simulink model "Commande"  (R2020b)
settings: Solver=VariableStepAuto  StartTime=0.0  StopTime=1  RelTol=1e-3
undefined symbols (not defined in the file or in its folder): FC, FuelCellLoadFcn, gcbh, ln, sps_rtmsupport, Ts
libraries: simulink x43, powerlib x37, powerlib_meascontrol x7, fuzblock x4, powerlib_extras x2
(part 3 of 3)

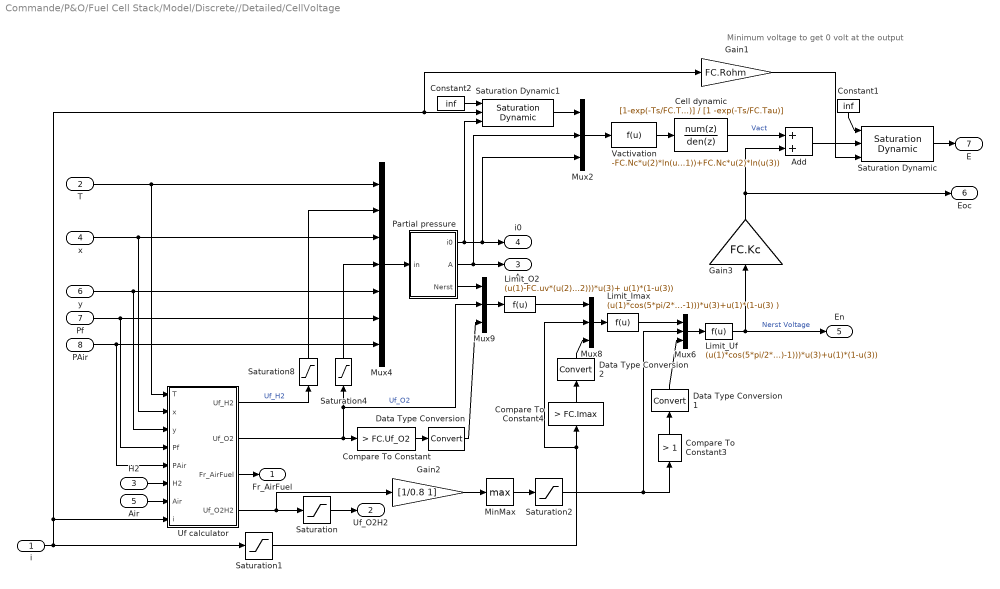
== system Commande/P&O/Fuel Cell Stack/Model/Discrete//Detailed/CellVoltage ==
  note: Minimum voltage to get 0 volt at the output
  i : Inport
  T : Inport  Port=2
  H2 : Inport  Port=3
  x : Inport  Port=4
  Air : Inport  Port=5
  y : Inport  Port=6
  Pf : Inport  Port=7
  PAir : Inport  Port=8
  Add : Sum
  Cell dynamic : DiscreteTransferFcn  Numerator=[1-exp(-Ts/FC.Tau)]  Denominator=[1 -exp(-Ts/FC.Tau)]  SampleTime=Ts
  Compare To Constant : simulink/Logic and Bit Operations/Compare To Constant  relop=>  const=FC.Uf_O2  OutDataTypeStr=boolean
  Compare To Constant3 : simulink/Logic and Bit Operations/Compare To Constant  relop=>  const=1  OutDataTypeStr=boolean
  Compare To Constant4 : simulink/Logic and Bit Operations/Compare To Constant  relop=>  const=FC.Imax  OutDataTypeStr=boolean
  Constant1 : Constant  Value=inf
  Constant2 : Constant  Value=inf
  Data Type Conversion : DataTypeConversion
  Data Type Conversion1 : DataTypeConversion
  Data Type Conversion2 : DataTypeConversion
  Gain1 : Gain  Gain=FC.Rohm
  Gain2 : Gain  Gain=[1/0.8 1]
  Gain3 : Gain  Gain=FC.Kc
  Limit_Imax : Fcn  Expr=(u(1)*cos(5*pi/2*(u(2)/FC.Imax-1)))*u(3)+u(1)*(1-u(3) )
  Limit_O2 : Fcn  Expr=(u(1)-FC.uv*(u(2)-FC.Uf_O2)/(FC.Kc*(FC.ufO2max-FC.Uf_O2)))*u(3)+ u(1)*(1-u(3))
  Limit_Uf : Fcn  Expr=(u(1)*cos(5*pi/2*(u(2)-1)))*u(3)+u(1)*(1-u(3))
  MinMax : MinMax  Function=max
  Mux{2,6,8..9} (4 alike) : Mux  Inputs=3
  Mux4 : Mux  Inputs=7
  Partial pressure : Subsystem
  Saturation : Saturate  UpperLimit=0.9999  LowerLimit=0.0001
  Saturation Dynamic : simulink/Discontinuities/Saturation Dynamic  OutMin=[]  OutMax=[]  OutDataTypeStr=Inherit: Same as second input  OutDataType=fixdt(1, 16)  OutScaling=2^-10  DoSatur=off
  Saturation Dynamic1 : simulink/Discontinuities/Saturation Dynamic  OutMin=[]  OutMax=[]  OutDataTypeStr=Inherit: Same as second input  OutDataType=fixdt(1, 16)  OutScaling=2^-10  DoSatur=off
  Saturation1 : Saturate  UpperLimit=FC.Imax*1.2  LowerLimit=0
  Saturation2 : Saturate  UpperLimit=1.2  LowerLimit=0
  Saturation4 : Saturate  UpperLimit=FC.Uf_O2  LowerLimit=0
  Saturation8 : Saturate  UpperLimit=FC.Uf_H2  LowerLimit=0
  Uf calculator : Subsystem
  Vactivation : Fcn  Expr=-FC.Nc*u(2)*ln(u(1))+FC.Nc*u(2)*ln(u(3))
  Fr_AirFuel : Outport  VectorParamsAs1DForOutWhenUnconnected=off
  Uf_O2H2 : Outport  Port=2  VectorParamsAs1DForOutWhenUnconnected=off
  A : Outport  Port=3  VectorParamsAs1DForOutWhenUnconnected=off
  i0 : Outport  Port=4  VectorParamsAs1DForOutWhenUnconnected=off
  En : Outport  Port=5  VectorParamsAs1DForOutWhenUnconnected=off
  Eoc : Outport  Port=6  VectorParamsAs1DForOutWhenUnconnected=off
  E : Outport  Port=7  VectorParamsAs1DForOutWhenUnconnected=off
  wires:
  Gain3/1 -> Eoc/1, Add/2
  T/1 -> Uf calculator/1(T), Mux4/1
  x/1 -> Mux4/3, Uf calculator/2(x)
  y/1 -> Mux4/5, Uf calculator/3(y)
  Pf/1 -> Mux4/6, Uf calculator/4(Pf)
  PAir/1 -> Mux4/7, Uf calculator/5(PAir)
  Partial pressure/1(i0) -> Saturation Dynamic1/3, i0/1, Mux2/3
  Partial pressure/2(A) -> A/1, Mux2/2
  H2/1 -> Uf calculator/6(H2)
  i/1 -> Uf calculator/8(i), Saturation Dynamic1/2, Gain1/1, Saturation1/1
  Uf calculator/1(Uf_H2) -> Saturation8/1  "Uf_H2"
  Uf calculator/2(Uf_O2) -> Compare To Constant/1, Saturation4/1, Mux9/2  "Uf_O2"
  Air/1 -> Uf calculator/7(Air)
  Mux8/1 -> Limit_Imax/1
  Limit_Imax/1 -> Mux6/1
  Limit_Uf/1 -> Gain3/1, En/1  "Nerst Voltage"
  Uf calculator/3(Fr_AirFuel) -> Fr_AirFuel/1
  Mux9/1 -> Limit_O2/1
  Limit_O2/1 -> Mux8/1
  Saturation8/1 -> Mux4/2
  Uf calculator/4(Uf_O2H2) -> Saturation/1, Gain2/1
  Mux4/1 -> Partial pressure/1(in)
  Constant2/1 -> Saturation Dynamic1/1
  Saturation Dynamic1/1 -> Mux2/1
  Mux2/1 -> Vactivation/1
  Vactivation/1 -> Cell dynamic/1
  Cell dynamic/1 -> Add/1  "Vact"
  Add/1 -> Saturation Dynamic/2
  Saturation Dynamic/1 -> E/1
  Constant1/1 -> Saturation Dynamic/1
  Gain1/1 -> Saturation Dynamic/3
  Mux6/1 -> Limit_Uf/1
  Saturation/1 -> Uf_O2H2/1
  MinMax/1 -> Saturation2/1
  Saturation4/1 -> Mux4/4
  Partial pressure/3(Nerst) -> Mux9/1
  Gain2/1 -> MinMax/1
  Compare To Constant/1 -> Data Type Conversion/1
  Data Type Conversion/1 -> Mux9/3
  Data Type Conversion2/1 -> Mux8/3
  Compare To Constant4/1 -> Data Type Conversion2/1
  Saturation1/1 -> Mux8/2, Compare To Constant4/1
  Saturation2/1 -> Mux6/2, Compare To Constant3/1
  Compare To Constant3/1 -> Data Type Conversion1/1
  Data Type Conversion1/1 -> Mux6/3

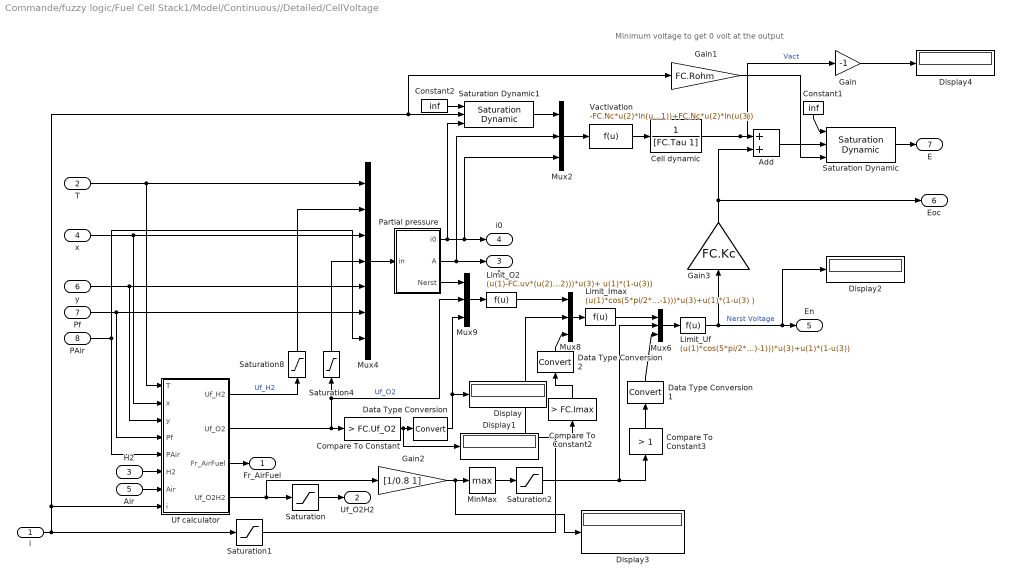
== system Commande/fuzzy logic/Fuel Cell Stack1/Model/Continuous//Detailed/CellVoltage ==
  note: Minimum voltage to get 0 volt at the output
  i : Inport
  T : Inport  Port=2
  H2 : Inport  Port=3
  x : Inport  Port=4
  Air : Inport  Port=5
  y : Inport  Port=6
  Pf : Inport  Port=7
  PAir : Inport  Port=8
  Add : Sum
  Cell dynamic : TransferFcn  Denominator=[FC.Tau 1]
  Compare To Constant : simulink/Logic and Bit Operations/Compare To Constant  relop=>  const=FC.Uf_O2  OutDataTypeStr=boolean
  Compare To Constant2 : simulink/Logic and Bit Operations/Compare To Constant  relop=>  const=FC.Imax  OutDataTypeStr=boolean
  Compare To Constant3 : simulink/Logic and Bit Operations/Compare To Constant  relop=>  const=1  OutDataTypeStr=boolean
  Constant1 : Constant  Value=inf
  Constant2 : Constant  Value=inf
  Data Type Conversion : DataTypeConversion
  Data Type Conversion1 : DataTypeConversion
  Data Type Conversion2 : DataTypeConversion
  Display{,1..4} (5 alike) : Display
  Gain : Gain  Gain=-1
  Gain1 : Gain  Gain=FC.Rohm
  Gain2 : Gain  Gain=[1/0.8 1]
  Gain3 : Gain  Gain=FC.Kc
  Limit_Imax : Fcn  Expr=(u(1)*cos(5*pi/2*(u(2)/FC.Imax-1)))*u(3)+u(1)*(1-u(3) )
  Limit_O2 : Fcn  Expr=(u(1)-FC.uv*(u(2)-FC.Uf_O2)/(FC.Kc*(FC.ufO2max-FC.Uf_O2)))*u(3)+ u(1)*(1-u(3))
  Limit_Uf : Fcn  Expr=(u(1)*cos(5*pi/2*(u(2)-1)))*u(3)+u(1)*(1-u(3))
  MinMax : MinMax  Function=max
  Mux{2,6,8..9} (4 alike) : Mux  Inputs=3
  Mux4 : Mux  Inputs=7
  Partial pressure : Subsystem
  Saturation : Saturate  UpperLimit=0.9999  LowerLimit=0.0001
  Saturation Dynamic : simulink/Discontinuities/Saturation Dynamic  OutMin=[]  OutMax=[]  OutDataTypeStr=Inherit: Same as second input  OutDataType=fixdt(1, 16)  OutScaling=2^-10  DoSatur=off
  Saturation Dynamic1 : simulink/Discontinuities/Saturation Dynamic  OutMin=[]  OutMax=[]  OutDataTypeStr=Inherit: Same as second input  OutDataType=fixdt(1, 16)  OutScaling=2^-10  DoSatur=off
  Saturation1 : Saturate  UpperLimit=FC.Imax*1.2  LowerLimit=0
  Saturation2 : Saturate  UpperLimit=1.2  LowerLimit=0
  Saturation4 : Saturate  UpperLimit=FC.Uf_O2  LowerLimit=0
  Saturation8 : Saturate  UpperLimit=FC.Uf_H2  LowerLimit=0
  Uf calculator : Subsystem
  Vactivation : Fcn  Expr=-FC.Nc*u(2)*ln(u(1))+FC.Nc*u(2)*ln(u(3))
  Fr_AirFuel : Outport  VectorParamsAs1DForOutWhenUnconnected=off
  Uf_O2H2 : Outport  Port=2  VectorParamsAs1DForOutWhenUnconnected=off
  A : Outport  Port=3  VectorParamsAs1DForOutWhenUnconnected=off
  i0 : Outport  Port=4  VectorParamsAs1DForOutWhenUnconnected=off
  En : Outport  Port=5  VectorParamsAs1DForOutWhenUnconnected=off
  Eoc : Outport  Port=6  VectorParamsAs1DForOutWhenUnconnected=off
  E : Outport  Port=7  VectorParamsAs1DForOutWhenUnconnected=off
  wires:
  Gain3/1 -> Eoc/1, Add/2
  Data Type Conversion1/1 -> Mux6/3
  Compare To Constant3/1 -> Data Type Conversion1/1
  Saturation2/1 -> Mux6/2, Compare To Constant3/1
  Saturation1/1 -> Mux8/2, Compare To Constant2/1
  Compare To Constant2/1 -> Data Type Conversion2/1
  Data Type Conversion2/1 -> Mux8/3
  Compare To Constant/1 -> Display1/1, Data Type Conversion/1
  Gain2/1 -> Display3/1, MinMax/1
  Partial pressure/3(Nerst) -> Mux9/1
  Saturation4/1 -> Mux4/4
  MinMax/1 -> Saturation2/1
  Saturation/1 -> Uf_O2H2/1
  Mux6/1 -> Limit_Uf/1
  Gain1/1 -> Saturation Dynamic/3
  Constant1/1 -> Saturation Dynamic/1
  Saturation Dynamic/1 -> E/1
  Add/1 -> Saturation Dynamic/2
  Cell dynamic/1 -> Gain/1, Add/1  "Vact"
  Vactivation/1 -> Cell dynamic/1
  Mux2/1 -> Vactivation/1
  Saturation Dynamic1/1 -> Mux2/1
  Constant2/1 -> Saturation Dynamic1/1
  Mux4/1 -> Partial pressure/1(in)
  Uf calculator/4(Uf_O2H2) -> Gain2/1, Saturation/1
  Saturation8/1 -> Mux4/2
  Limit_O2/1 -> Mux8/1
  Mux9/1 -> Limit_O2/1
  Uf calculator/3(Fr_AirFuel) -> Fr_AirFuel/1
  Limit_Uf/1 -> Gain3/1, Display2/1, En/1  "Nerst Voltage"
  Limit_Imax/1 -> Mux6/1
  Mux8/1 -> Limit_Imax/1
  Air/1 -> Uf calculator/7(Air)
  Uf calculator/2(Uf_O2) -> Mux9/2, Saturation4/1, Compare To Constant/1  "Uf_O2"
  Uf calculator/1(Uf_H2) -> Saturation8/1  "Uf_H2"
  i/1 -> Saturation1/1, Uf calculator/8(i), Gain1/1, Saturation Dynamic1/2
  H2/1 -> Uf calculator/6(H2)
  Partial pressure/2(A) -> Mux2/2, A/1
  Partial pressure/1(i0) -> Mux2/3, i0/1, Saturation Dynamic1/3
  PAir/1 -> Uf calculator/5(PAir), Mux4/7
  Pf/1 -> Uf calculator/4(Pf), Mux4/6
  y/1 -> Uf calculator/3(y), Mux4/5
  x/1 -> Uf calculator/2(x), Mux4/3
  T/1 -> Uf calculator/1(T), Mux4/1
  Data Type Conversion/1 -> Display/1, Mux9/3
  Gain/1 -> Display4/1

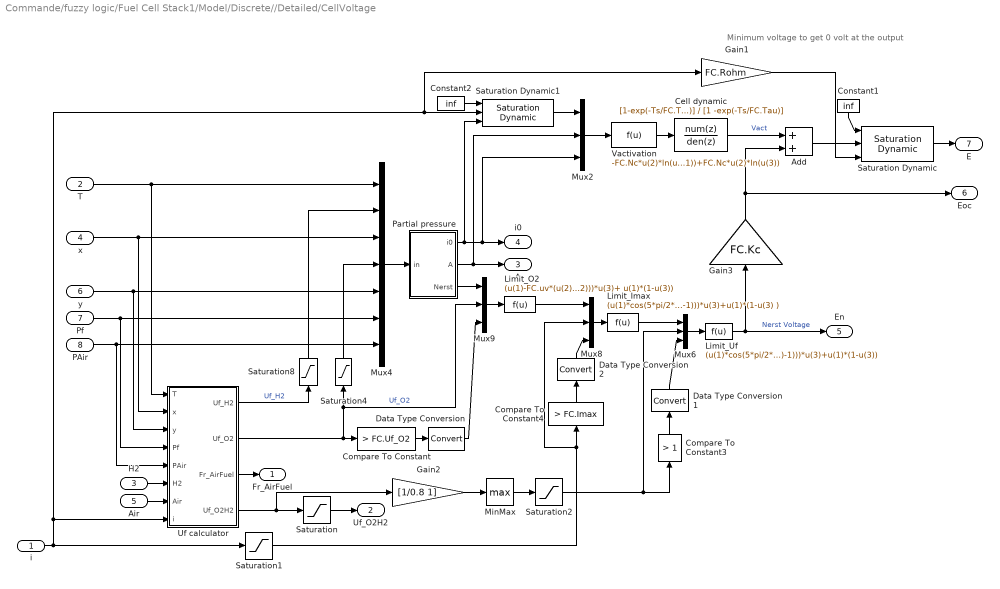
== system Commande/fuzzy logic/Fuel Cell Stack1/Model/Discrete//Detailed/CellVoltage ==
  note: Minimum voltage to get 0 volt at the output
  i : Inport
  T : Inport  Port=2
  H2 : Inport  Port=3
  x : Inport  Port=4
  Air : Inport  Port=5
  y : Inport  Port=6
  Pf : Inport  Port=7
  PAir : Inport  Port=8
  Add : Sum
  Cell dynamic : DiscreteTransferFcn  Numerator=[1-exp(-Ts/FC.Tau)]  Denominator=[1 -exp(-Ts/FC.Tau)]  SampleTime=Ts
  Compare To Constant : simulink/Logic and Bit Operations/Compare To Constant  relop=>  const=FC.Uf_O2  OutDataTypeStr=boolean
  Compare To Constant3 : simulink/Logic and Bit Operations/Compare To Constant  relop=>  const=1  OutDataTypeStr=boolean
  Compare To Constant4 : simulink/Logic and Bit Operations/Compare To Constant  relop=>  const=FC.Imax  OutDataTypeStr=boolean
  Constant1 : Constant  Value=inf
  Constant2 : Constant  Value=inf
  Data Type Conversion : DataTypeConversion
  Data Type Conversion1 : DataTypeConversion
  Data Type Conversion2 : DataTypeConversion
  Gain1 : Gain  Gain=FC.Rohm
  Gain2 : Gain  Gain=[1/0.8 1]
  Gain3 : Gain  Gain=FC.Kc
  Limit_Imax : Fcn  Expr=(u(1)*cos(5*pi/2*(u(2)/FC.Imax-1)))*u(3)+u(1)*(1-u(3) )
  Limit_O2 : Fcn  Expr=(u(1)-FC.uv*(u(2)-FC.Uf_O2)/(FC.Kc*(FC.ufO2max-FC.Uf_O2)))*u(3)+ u(1)*(1-u(3))
  Limit_Uf : Fcn  Expr=(u(1)*cos(5*pi/2*(u(2)-1)))*u(3)+u(1)*(1-u(3))
  MinMax : MinMax  Function=max
  Mux{2,6,8..9} (4 alike) : Mux  Inputs=3
  Mux4 : Mux  Inputs=7
  Partial pressure : Subsystem
  Saturation : Saturate  UpperLimit=0.9999  LowerLimit=0.0001
  Saturation Dynamic : simulink/Discontinuities/Saturation Dynamic  OutMin=[]  OutMax=[]  OutDataTypeStr=Inherit: Same as second input  OutDataType=fixdt(1, 16)  OutScaling=2^-10  DoSatur=off
  Saturation Dynamic1 : simulink/Discontinuities/Saturation Dynamic  OutMin=[]  OutMax=[]  OutDataTypeStr=Inherit: Same as second input  OutDataType=fixdt(1, 16)  OutScaling=2^-10  DoSatur=off
  Saturation1 : Saturate  UpperLimit=FC.Imax*1.2  LowerLimit=0
  Saturation2 : Saturate  UpperLimit=1.2  LowerLimit=0
  Saturation4 : Saturate  UpperLimit=FC.Uf_O2  LowerLimit=0
  Saturation8 : Saturate  UpperLimit=FC.Uf_H2  LowerLimit=0
  Uf calculator : Subsystem
  Vactivation : Fcn  Expr=-FC.Nc*u(2)*ln(u(1))+FC.Nc*u(2)*ln(u(3))
  Fr_AirFuel : Outport  VectorParamsAs1DForOutWhenUnconnected=off
  Uf_O2H2 : Outport  Port=2  VectorParamsAs1DForOutWhenUnconnected=off
  A : Outport  Port=3  VectorParamsAs1DForOutWhenUnconnected=off
  i0 : Outport  Port=4  VectorParamsAs1DForOutWhenUnconnected=off
  En : Outport  Port=5  VectorParamsAs1DForOutWhenUnconnected=off
  Eoc : Outport  Port=6  VectorParamsAs1DForOutWhenUnconnected=off
  E : Outport  Port=7  VectorParamsAs1DForOutWhenUnconnected=off
  wires:
  Gain3/1 -> Eoc/1, Add/2
  T/1 -> Uf calculator/1(T), Mux4/1
  x/1 -> Mux4/3, Uf calculator/2(x)
  y/1 -> Mux4/5, Uf calculator/3(y)
  Pf/1 -> Mux4/6, Uf calculator/4(Pf)
  PAir/1 -> Mux4/7, Uf calculator/5(PAir)
  Partial pressure/1(i0) -> Saturation Dynamic1/3, i0/1, Mux2/3
  Partial pressure/2(A) -> A/1, Mux2/2
  H2/1 -> Uf calculator/6(H2)
  i/1 -> Uf calculator/8(i), Saturation Dynamic1/2, Gain1/1, Saturation1/1
  Uf calculator/1(Uf_H2) -> Saturation8/1  "Uf_H2"
  Uf calculator/2(Uf_O2) -> Compare To Constant/1, Saturation4/1, Mux9/2  "Uf_O2"
  Air/1 -> Uf calculator/7(Air)
  Mux8/1 -> Limit_Imax/1
  Limit_Imax/1 -> Mux6/1
  Limit_Uf/1 -> Gain3/1, En/1  "Nerst Voltage"
  Uf calculator/3(Fr_AirFuel) -> Fr_AirFuel/1
  Mux9/1 -> Limit_O2/1
  Limit_O2/1 -> Mux8/1
  Saturation8/1 -> Mux4/2
  Uf calculator/4(Uf_O2H2) -> Saturation/1, Gain2/1
  Mux4/1 -> Partial pressure/1(in)
  Constant2/1 -> Saturation Dynamic1/1
  Saturation Dynamic1/1 -> Mux2/1
  Mux2/1 -> Vactivation/1
  Vactivation/1 -> Cell dynamic/1
  Cell dynamic/1 -> Add/1  "Vact"
  Add/1 -> Saturation Dynamic/2
  Saturation Dynamic/1 -> E/1
  Constant1/1 -> Saturation Dynamic/1
  Gain1/1 -> Saturation Dynamic/3
  Mux6/1 -> Limit_Uf/1
  Saturation/1 -> Uf_O2H2/1
  MinMax/1 -> Saturation2/1
  Saturation4/1 -> Mux4/4
  Partial pressure/3(Nerst) -> Mux9/1
  Gain2/1 -> MinMax/1
  Compare To Constant/1 -> Data Type Conversion/1
  Data Type Conversion/1 -> Mux9/3
  Data Type Conversion2/1 -> Mux8/3
  Compare To Constant4/1 -> Data Type Conversion2/1
  Saturation1/1 -> Mux8/2, Compare To Constant4/1
  Saturation2/1 -> Mux6/2, Compare To Constant3/1
  Compare To Constant3/1 -> Data Type Conversion1/1
  Data Type Conversion1/1 -> Mux6/3

== system Commande/INC 1/Fuel Cell Stack/Model/Continuous//Detailed/CellVoltage/Partial pressure ==
  in : Inport
  A2 : Fcn  Expr=(FC.R*u(1))/(2*FC.alpha*FC.F)
  Constant : Constant
  Cr : Fcn  Expr=(u(2)*FC.Pstd+u(3)*FC.Pstd)/(FC.R*u(1))
  Display : Display
  Display1 : Display
  Mux1 : Mux  Inputs=2
  Mux2 : Mux
  Nerst Voltage : Fcn  Expr=1.229+(u(1)-298.15)*(-44.43/(FC.z*FC.F))+(FC.R*u(1)/(FC.z*FC.F))*(log(u(2)*sqrt(u(3))/u(4)))
  PH2 : Fcn  Expr=u(3)*(1-u(2))*u(6)
  PH2O : Fcn  Expr=(FC.xy+2*u(5)*u(4))*u(7)
  PO2 : Fcn  Expr=u(5)*(1-u(4))*u(7)
  Saturation1 : Saturate  UpperLimit=inf  LowerLimit=0.0001
  Saturation4 : Saturate  UpperLimit=inf  LowerLimit=0.0001
  Saturation5 : Saturate  UpperLimit=inf  LowerLimit=0.0001
  Switch : Switch  Threshold=273+100
  Temp : Fcn  Expr=u(1)
  i0 calc : Fcn  Expr=2*FC.F*FC.k*u(1)*u(2)*exp(-FC.Dg/(FC.R*u(1)))/FC.h
  i0 : Outport  VectorParamsAs1DForOutWhenUnconnected=off
  A : Outport  Port=2  VectorParamsAs1DForOutWhenUnconnected=off
  Nerst : Outport  Port=3  VectorParamsAs1DForOutWhenUnconnected=off
  wires:
  Temp/1 -> Mux2/1, Switch/2, A2/1, Mux1/1
  i0 calc/1 -> i0/1
  Nerst Voltage/1 -> Display1/1, Nerst/1
  A2/1 -> A/1
  PH2O/1 -> Saturation5/1
  PO2/1 -> Saturation4/1
  PH2/1 -> Saturation1/1
  Saturation1/1 -> Mux2/2
  Saturation4/1 -> Mux2/3
  Switch/1 -> Mux2/4
  Saturation5/1 -> Switch/1
  Constant/1 -> Switch/3
  Mux2/1 -> Nerst Voltage/1, Cr/1
  in/1 -> PH2O/1, Display/1, Temp/1, PH2/1, PO2/1
  Mux1/1 -> i0 calc/1
  Cr/1 -> Mux1/2

== system Commande/INC 1/Fuel Cell Stack/Model/Continuous//Detailed/CellVoltage/Uf calculator ==
  T : Inport
  x : Inport  Port=2
  y : Inport  Port=3
  Pf : Inport  Port=4
  PAir : Inport  Port=5
  H2 : Inport  Port=6
  Air : Inport  Port=7
  i : Inport  Port=8
  AIR_flow_rate : Display
  Compare To Zero : simulink/Logic and Bit Operations/Compare To Zero  relop=>  OutDataTypeStr=uint8
  Constant : Constant  Value=FC.R
  Constant1 : Constant  Value=FC.sel_UfH2
  Constant2 : Constant  Value=FC.sel_UfO2
  Gain : Gain
  H2 utilization Fuel flowrate : Fcn  Expr=60000*FC.Nc*u(2)*FC.R*u(5)/(FC.z*FC.F*u(4)*FC.Pstd*u(3)*u(1))
  H2_airflow1 : Display
  Mux1 : Mux  Inputs=5
  Mux5 : Mux  Inputs=5
  Mux6 : Mux  Inputs=2
  Mux7 : Mux  Inputs=2
  O2 utilization Air flowrate : Fcn  Expr=60000*FC.Nc*u(2)*FC.R*u(5)/(4*FC.F*u(4)*FC.Pstd*u(3)*u(1))
  P_air : Display
  P_fuel : Display
  Product2 : Product  RndMeth=Zero
  Saturation3 : Saturate  UpperLimit=inf  LowerLimit=FC.AirFr_Max*0.01
  Switch{1..4} (4 alike) : Switch  Criteria=u2 > Threshold  Threshold=0.5
  UF_H2 : Display
  UF_O2 : Display
  X : Display
  Y : Display
  i_current : Display
  i_current1 : Display
  i_current2 : Display
  Uf_H2 : Outport  VectorParamsAs1DForOutWhenUnconnected=off
  Uf_O2 : Outport  Port=2  VectorParamsAs1DForOutWhenUnconnected=off
  Fr_AirFuel : Outport  Port=3  VectorParamsAs1DForOutWhenUnconnected=off
  Uf_O2H2 : Outport  Port=4  VectorParamsAs1DForOutWhenUnconnected=off
  wires:
  Switch1/1 -> Mux7/2, UF_H2/1, Uf_H2/1
  Saturation3/1 -> Mux5/3
  Switch2/1 -> Mux7/1, UF_O2/1, Uf_O2/1  "Uf_O2"
  Gain/1 -> Fr_AirFuel/1
  Switch4/1 -> Mux6/1
  Switch3/1 -> Mux6/2
  Mux6/1 -> Gain/1
  Pf/1 -> P_fuel/1, Mux1/4
  T/1 -> i_current2/1, Mux1/5, Mux5/5
  O2 utilization Air flowrate/1 -> Switch4/1, Switch2/3
  Constant2/1 -> Switch2/2, Switch4/2
  Constant1/1 -> Switch3/2, Switch1/2
  H2 utilization Fuel flowrate/1 -> Switch3/1, Switch1/3
  i/1 -> i_current/1, Compare To Zero/1, Mux1/2, i_current1/1, Mux5/2
  Air/1 -> AIR_flow_rate/1, Switch2/1, Switch4/3, Saturation3/1
  y/1 -> Y/1, Mux5/1
  H2/1 -> H2_airflow1/1, Mux1/3, Switch1/1, Switch3/3
  x/1 -> X/1, Mux1/1
  Mux5/1 -> O2 utilization Air flowrate/1
  Mux1/1 -> H2 utilization Fuel flowrate/1
  Mux7/1 -> Product2/2
  Product2/1 -> Uf_O2H2/1
  Compare To Zero/1 -> Product2/1
  PAir/1 -> P_air/1, Mux5/4

== system Commande/INC 1/Fuel Cell Stack/Model/Discrete//Detailed/CellVoltage/Partial pressure ==
  in : Inport
  A2 : Fcn  Expr=(FC.R*u(1))/(2*FC.alpha*FC.F)
  Constant : Constant
  Cr : Fcn  Expr=(u(2)*FC.Pstd+u(3)*FC.Pstd)/(FC.R*u(1))
  Mux1 : Mux  Inputs=2
  Mux2 : Mux
  Nerst Voltage : Fcn  Expr=1.229+(u(1)-298.15)*(-44.43/(FC.z*FC.F))+(FC.R*u(1)/(FC.z*FC.F))*(log(u(2)*sqrt(u(3))/u(4)))
  PH2 : Fcn  Expr=u(3)*(1-u(2))*u(6)
  PH2O : Fcn  Expr=(FC.xy+2*u(5)*u(4))*u(7)
  PO2 : Fcn  Expr=u(5)*(1-u(4))*u(7)
  Saturation1 : Saturate  UpperLimit=inf  LowerLimit=0.0001
  Saturation4 : Saturate  UpperLimit=inf  LowerLimit=0.0001
  Saturation5 : Saturate  UpperLimit=inf  LowerLimit=0.0001
  Switch : Switch  Threshold=273+100
  Temp : Fcn  Expr=u(1)
  i0 calc : Fcn  Expr=2*FC.F*FC.k*u(1)*u(2)*exp(-FC.Dg/(FC.R*u(1)))/FC.h
  i0 : Outport  VectorParamsAs1DForOutWhenUnconnected=off
  A : Outport  Port=2  VectorParamsAs1DForOutWhenUnconnected=off
  Nerst : Outport  Port=3  VectorParamsAs1DForOutWhenUnconnected=off
  wires:
  Cr/1 -> Mux1/2
  Mux1/1 -> i0 calc/1
  in/1 -> PO2/1, PH2/1, Temp/1, PH2O/1
  Mux2/1 -> Cr/1, Nerst Voltage/1
  Constant/1 -> Switch/3
  Saturation5/1 -> Switch/1
  Switch/1 -> Mux2/4
  Saturation4/1 -> Mux2/3
  Saturation1/1 -> Mux2/2
  PH2/1 -> Saturation1/1
  PO2/1 -> Saturation4/1
  PH2O/1 -> Saturation5/1
  A2/1 -> A/1
  Nerst Voltage/1 -> Nerst/1
  i0 calc/1 -> i0/1
  Temp/1 -> Mux1/1, A2/1, Switch/2, Mux2/1

== system Commande/INC 1/Fuel Cell Stack/Model/Discrete//Detailed/CellVoltage/Uf calculator ==
  T : Inport
  x : Inport  Port=2
  y : Inport  Port=3
  Pf : Inport  Port=4
  PAir : Inport  Port=5
  H2 : Inport  Port=6
  Air : Inport  Port=7
  i : Inport  Port=8
  Compare To Zero : simulink/Logic and Bit Operations/Compare To Zero  relop=>  OutDataTypeStr=uint8
  Constant1 : Constant  Value=FC.sel_UfH2
  Constant2 : Constant  Value=FC.sel_UfO2
  Gain : Gain
  H2 utilization Fuel flowrate : Fcn  Expr=60000*FC.Nc*u(2)*FC.R*u(5)/(FC.z*FC.F*u(4)*FC.Pstd*u(3)*u(1))
  Mux1 : Mux  Inputs=5
  Mux5 : Mux  Inputs=5
  Mux6 : Mux  Inputs=2
  Mux7 : Mux  Inputs=2
  O2 utilization Air flowrate : Fcn  Expr=60000*FC.Nc*u(2)*FC.R*u(5)/(4*FC.F*u(4)*FC.Pstd*u(3)*u(1))
  Product2 : Product  RndMeth=Zero
  Saturation3 : Saturate  UpperLimit=inf  LowerLimit=FC.AirFr_Max*0.01
  Switch{1..4} (4 alike) : Switch  Criteria=u2 > Threshold  Threshold=0.5
  Uf_H2 : Outport  VectorParamsAs1DForOutWhenUnconnected=off
  Uf_O2 : Outport  Port=2  VectorParamsAs1DForOutWhenUnconnected=off
  Fr_AirFuel : Outport  Port=3  VectorParamsAs1DForOutWhenUnconnected=off
  Uf_O2H2 : Outport  Port=4  VectorParamsAs1DForOutWhenUnconnected=off
  wires:
  Compare To Zero/1 -> Product2/1
  Product2/1 -> Uf_O2H2/1
  Mux7/1 -> Product2/2
  Mux1/1 -> H2 utilization Fuel flowrate/1
  Mux5/1 -> O2 utilization Air flowrate/1
  x/1 -> Mux1/1
  H2/1 -> Switch3/3, Switch1/1, Mux1/3
  y/1 -> Mux5/1
  Air/1 -> Switch4/3, Switch2/1, Saturation3/1
  i/1 -> Mux5/2, Mux1/2, Compare To Zero/1
  H2 utilization Fuel flowrate/1 -> Switch1/3, Switch3/1
  Constant1/1 -> Switch1/2, Switch3/2
  Constant2/1 -> Switch2/2, Switch4/2
  O2 utilization Air flowrate/1 -> Switch2/3, Switch4/1
  T/1 -> Mux5/5, Mux1/5
  Pf/1 -> Mux1/4
  PAir/1 -> Mux5/4
  Mux6/1 -> Gain/1
  Switch3/1 -> Mux6/2
  Switch4/1 -> Mux6/1
  Gain/1 -> Fr_AirFuel/1
  Switch2/1 -> Uf_O2/1, Mux7/1  "Uf_O2"
  Saturation3/1 -> Mux5/3
  Switch1/1 -> Uf_H2/1, Mux7/2

== system Commande/P&O/Fuel Cell Stack/Model/Continuous//Detailed/CellVoltage/Partial pressure ==
  in : Inport
  A2 : Fcn  Expr=(FC.R*u(1))/(2*FC.alpha*FC.F)
  Constant : Constant
  Cr : Fcn  Expr=(u(2)*FC.Pstd+u(3)*FC.Pstd)/(FC.R*u(1))
  Display : Display
  Display1 : Display
  Mux1 : Mux  Inputs=2
  Mux2 : Mux
  Nerst Voltage : Fcn  Expr=1.229+(u(1)-298.15)*(-44.43/(FC.z*FC.F))+(FC.R*u(1)/(FC.z*FC.F))*(log(u(2)*sqrt(u(3))/u(4)))
  PH2 : Fcn  Expr=u(3)*(1-u(2))*u(6)
  PH2O : Fcn  Expr=(FC.xy+2*u(5)*u(4))*u(7)
  PO2 : Fcn  Expr=u(5)*(1-u(4))*u(7)
  Saturation1 : Saturate  UpperLimit=inf  LowerLimit=0.0001
  Saturation4 : Saturate  UpperLimit=inf  LowerLimit=0.0001
  Saturation5 : Saturate  UpperLimit=inf  LowerLimit=0.0001
  Switch : Switch  Threshold=273+100
  Temp : Fcn  Expr=u(1)
  i0 calc : Fcn  Expr=2*FC.F*FC.k*u(1)*u(2)*exp(-FC.Dg/(FC.R*u(1)))/FC.h
  i0 : Outport  VectorParamsAs1DForOutWhenUnconnected=off
  A : Outport  Port=2  VectorParamsAs1DForOutWhenUnconnected=off
  Nerst : Outport  Port=3  VectorParamsAs1DForOutWhenUnconnected=off
  wires:
  Temp/1 -> Mux2/1, Switch/2, A2/1, Mux1/1
  i0 calc/1 -> i0/1
  Nerst Voltage/1 -> Display1/1, Nerst/1
  A2/1 -> A/1
  PH2O/1 -> Saturation5/1
  PO2/1 -> Saturation4/1
  PH2/1 -> Saturation1/1
  Saturation1/1 -> Mux2/2
  Saturation4/1 -> Mux2/3
  Switch/1 -> Mux2/4
  Saturation5/1 -> Switch/1
  Constant/1 -> Switch/3
  Mux2/1 -> Nerst Voltage/1, Cr/1
  in/1 -> PH2O/1, Display/1, Temp/1, PH2/1, PO2/1
  Mux1/1 -> i0 calc/1
  Cr/1 -> Mux1/2

== system Commande/P&O/Fuel Cell Stack/Model/Continuous//Detailed/CellVoltage/Uf calculator ==
  T : Inport
  x : Inport  Port=2
  y : Inport  Port=3
  Pf : Inport  Port=4
  PAir : Inport  Port=5
  H2 : Inport  Port=6
  Air : Inport  Port=7
  i : Inport  Port=8
  AIR_flow_rate : Display
  Compare To Zero : simulink/Logic and Bit Operations/Compare To Zero  relop=>  OutDataTypeStr=uint8
  Constant : Constant  Value=FC.R
  Constant1 : Constant  Value=FC.sel_UfH2
  Constant2 : Constant  Value=FC.sel_UfO2
  Gain : Gain
  H2 utilization Fuel flowrate : Fcn  Expr=60000*FC.Nc*u(2)*FC.R*u(5)/(FC.z*FC.F*u(4)*FC.Pstd*u(3)*u(1))
  H2_airflow1 : Display
  Mux1 : Mux  Inputs=5
  Mux5 : Mux  Inputs=5
  Mux6 : Mux  Inputs=2
  Mux7 : Mux  Inputs=2
  O2 utilization Air flowrate : Fcn  Expr=60000*FC.Nc*u(2)*FC.R*u(5)/(4*FC.F*u(4)*FC.Pstd*u(3)*u(1))
  P_air : Display
  P_fuel : Display
  Product2 : Product  RndMeth=Zero
  Saturation3 : Saturate  UpperLimit=inf  LowerLimit=FC.AirFr_Max*0.01
  Switch{1..4} (4 alike) : Switch  Criteria=u2 > Threshold  Threshold=0.5
  UF_H2 : Display
  UF_O2 : Display
  X : Display
  Y : Display
  i_current : Display
  i_current1 : Display
  i_current2 : Display
  Uf_H2 : Outport  VectorParamsAs1DForOutWhenUnconnected=off
  Uf_O2 : Outport  Port=2  VectorParamsAs1DForOutWhenUnconnected=off
  Fr_AirFuel : Outport  Port=3  VectorParamsAs1DForOutWhenUnconnected=off
  Uf_O2H2 : Outport  Port=4  VectorParamsAs1DForOutWhenUnconnected=off
  wires:
  Switch1/1 -> Mux7/2, UF_H2/1, Uf_H2/1
  Saturation3/1 -> Mux5/3
  Switch2/1 -> Mux7/1, UF_O2/1, Uf_O2/1  "Uf_O2"
  Gain/1 -> Fr_AirFuel/1
  Switch4/1 -> Mux6/1
  Switch3/1 -> Mux6/2
  Mux6/1 -> Gain/1
  Pf/1 -> P_fuel/1, Mux1/4
  T/1 -> i_current2/1, Mux1/5, Mux5/5
  O2 utilization Air flowrate/1 -> Switch4/1, Switch2/3
  Constant2/1 -> Switch2/2, Switch4/2
  Constant1/1 -> Switch3/2, Switch1/2
  H2 utilization Fuel flowrate/1 -> Switch3/1, Switch1/3
  i/1 -> i_current/1, Compare To Zero/1, Mux1/2, i_current1/1, Mux5/2
  Air/1 -> AIR_flow_rate/1, Switch2/1, Switch4/3, Saturation3/1
  y/1 -> Y/1, Mux5/1
  H2/1 -> H2_airflow1/1, Mux1/3, Switch1/1, Switch3/3
  x/1 -> X/1, Mux1/1
  Mux5/1 -> O2 utilization Air flowrate/1
  Mux1/1 -> H2 utilization Fuel flowrate/1
  Mux7/1 -> Product2/2
  Product2/1 -> Uf_O2H2/1
  Compare To Zero/1 -> Product2/1
  PAir/1 -> P_air/1, Mux5/4

== system Commande/P&O/Fuel Cell Stack/Model/Discrete//Detailed/CellVoltage/Partial pressure ==
  in : Inport
  A2 : Fcn  Expr=(FC.R*u(1))/(2*FC.alpha*FC.F)
  Constant : Constant
  Cr : Fcn  Expr=(u(2)*FC.Pstd+u(3)*FC.Pstd)/(FC.R*u(1))
  Mux1 : Mux  Inputs=2
  Mux2 : Mux
  Nerst Voltage : Fcn  Expr=1.229+(u(1)-298.15)*(-44.43/(FC.z*FC.F))+(FC.R*u(1)/(FC.z*FC.F))*(log(u(2)*sqrt(u(3))/u(4)))
  PH2 : Fcn  Expr=u(3)*(1-u(2))*u(6)
  PH2O : Fcn  Expr=(FC.xy+2*u(5)*u(4))*u(7)
  PO2 : Fcn  Expr=u(5)*(1-u(4))*u(7)
  Saturation1 : Saturate  UpperLimit=inf  LowerLimit=0.0001
  Saturation4 : Saturate  UpperLimit=inf  LowerLimit=0.0001
  Saturation5 : Saturate  UpperLimit=inf  LowerLimit=0.0001
  Switch : Switch  Threshold=273+100
  Temp : Fcn  Expr=u(1)
  i0 calc : Fcn  Expr=2*FC.F*FC.k*u(1)*u(2)*exp(-FC.Dg/(FC.R*u(1)))/FC.h
  i0 : Outport  VectorParamsAs1DForOutWhenUnconnected=off
  A : Outport  Port=2  VectorParamsAs1DForOutWhenUnconnected=off
  Nerst : Outport  Port=3  VectorParamsAs1DForOutWhenUnconnected=off
  wires:
  Cr/1 -> Mux1/2
  Mux1/1 -> i0 calc/1
  in/1 -> PO2/1, PH2/1, Temp/1, PH2O/1
  Mux2/1 -> Cr/1, Nerst Voltage/1
  Constant/1 -> Switch/3
  Saturation5/1 -> Switch/1
  Switch/1 -> Mux2/4
  Saturation4/1 -> Mux2/3
  Saturation1/1 -> Mux2/2
  PH2/1 -> Saturation1/1
  PO2/1 -> Saturation4/1
  PH2O/1 -> Saturation5/1
  A2/1 -> A/1
  Nerst Voltage/1 -> Nerst/1
  i0 calc/1 -> i0/1
  Temp/1 -> Mux1/1, A2/1, Switch/2, Mux2/1

== system Commande/P&O/Fuel Cell Stack/Model/Discrete//Detailed/CellVoltage/Uf calculator ==
  T : Inport
  x : Inport  Port=2
  y : Inport  Port=3
  Pf : Inport  Port=4
  PAir : Inport  Port=5
  H2 : Inport  Port=6
  Air : Inport  Port=7
  i : Inport  Port=8
  Compare To Zero : simulink/Logic and Bit Operations/Compare To Zero  relop=>  OutDataTypeStr=uint8
  Constant1 : Constant  Value=FC.sel_UfH2
  Constant2 : Constant  Value=FC.sel_UfO2
  Gain : Gain
  H2 utilization Fuel flowrate : Fcn  Expr=60000*FC.Nc*u(2)*FC.R*u(5)/(FC.z*FC.F*u(4)*FC.Pstd*u(3)*u(1))
  Mux1 : Mux  Inputs=5
  Mux5 : Mux  Inputs=5
  Mux6 : Mux  Inputs=2
  Mux7 : Mux  Inputs=2
  O2 utilization Air flowrate : Fcn  Expr=60000*FC.Nc*u(2)*FC.R*u(5)/(4*FC.F*u(4)*FC.Pstd*u(3)*u(1))
  Product2 : Product  RndMeth=Zero
  Saturation3 : Saturate  UpperLimit=inf  LowerLimit=FC.AirFr_Max*0.01
  Switch{1..4} (4 alike) : Switch  Criteria=u2 > Threshold  Threshold=0.5
  Uf_H2 : Outport  VectorParamsAs1DForOutWhenUnconnected=off
  Uf_O2 : Outport  Port=2  VectorParamsAs1DForOutWhenUnconnected=off
  Fr_AirFuel : Outport  Port=3  VectorParamsAs1DForOutWhenUnconnected=off
  Uf_O2H2 : Outport  Port=4  VectorParamsAs1DForOutWhenUnconnected=off
  wires:
  Compare To Zero/1 -> Product2/1
  Product2/1 -> Uf_O2H2/1
  Mux7/1 -> Product2/2
  Mux1/1 -> H2 utilization Fuel flowrate/1
  Mux5/1 -> O2 utilization Air flowrate/1
  x/1 -> Mux1/1
  H2/1 -> Switch3/3, Switch1/1, Mux1/3
  y/1 -> Mux5/1
  Air/1 -> Switch4/3, Switch2/1, Saturation3/1
  i/1 -> Mux5/2, Mux1/2, Compare To Zero/1
  H2 utilization Fuel flowrate/1 -> Switch1/3, Switch3/1
  Constant1/1 -> Switch1/2, Switch3/2
  Constant2/1 -> Switch2/2, Switch4/2
  O2 utilization Air flowrate/1 -> Switch2/3, Switch4/1
  T/1 -> Mux5/5, Mux1/5
  Pf/1 -> Mux1/4
  PAir/1 -> Mux5/4
  Mux6/1 -> Gain/1
  Switch3/1 -> Mux6/2
  Switch4/1 -> Mux6/1
  Gain/1 -> Fr_AirFuel/1
  Switch2/1 -> Uf_O2/1, Mux7/1  "Uf_O2"
  Saturation3/1 -> Mux5/3
  Switch1/1 -> Uf_H2/1, Mux7/2

== system Commande/fuzzy logic/Fuel Cell Stack1/Model/Continuous//Detailed/CellVoltage/Partial pressure ==
  in : Inport
  A2 : Fcn  Expr=(FC.R*u(1))/(2*FC.alpha*FC.F)
  Constant : Constant
  Cr : Fcn  Expr=(u(2)*FC.Pstd+u(3)*FC.Pstd)/(FC.R*u(1))
  Display : Display
  Display1 : Display
  Mux1 : Mux  Inputs=2
  Mux2 : Mux
  Nerst Voltage : Fcn  Expr=1.229+(u(1)-298.15)*(-44.43/(FC.z*FC.F))+(FC.R*u(1)/(FC.z*FC.F))*(log(u(2)*sqrt(u(3))/u(4)))
  PH2 : Fcn  Expr=u(3)*(1-u(2))*u(6)
  PH2O : Fcn  Expr=(FC.xy+2*u(5)*u(4))*u(7)
  PO2 : Fcn  Expr=u(5)*(1-u(4))*u(7)
  Saturation1 : Saturate  UpperLimit=inf  LowerLimit=0.0001
  Saturation4 : Saturate  UpperLimit=inf  LowerLimit=0.0001
  Saturation5 : Saturate  UpperLimit=inf  LowerLimit=0.0001
  Switch : Switch  Threshold=273+100
  Temp : Fcn  Expr=u(1)
  i0 calc : Fcn  Expr=2*FC.F*FC.k*u(1)*u(2)*exp(-FC.Dg/(FC.R*u(1)))/FC.h
  i0 : Outport  VectorParamsAs1DForOutWhenUnconnected=off
  A : Outport  Port=2  VectorParamsAs1DForOutWhenUnconnected=off
  Nerst : Outport  Port=3  VectorParamsAs1DForOutWhenUnconnected=off
  wires:
  Temp/1 -> Mux2/1, Switch/2, A2/1, Mux1/1
  i0 calc/1 -> i0/1
  Nerst Voltage/1 -> Display1/1, Nerst/1
  A2/1 -> A/1
  PH2O/1 -> Saturation5/1
  PO2/1 -> Saturation4/1
  PH2/1 -> Saturation1/1
  Saturation1/1 -> Mux2/2
  Saturation4/1 -> Mux2/3
  Switch/1 -> Mux2/4
  Saturation5/1 -> Switch/1
  Constant/1 -> Switch/3
  Mux2/1 -> Nerst Voltage/1, Cr/1
  in/1 -> PH2O/1, Display/1, Temp/1, PH2/1, PO2/1
  Mux1/1 -> i0 calc/1
  Cr/1 -> Mux1/2

== system Commande/fuzzy logic/Fuel Cell Stack1/Model/Continuous//Detailed/CellVoltage/Uf calculator ==
  T : Inport
  x : Inport  Port=2
  y : Inport  Port=3
  Pf : Inport  Port=4
  PAir : Inport  Port=5
  H2 : Inport  Port=6
  Air : Inport  Port=7
  i : Inport  Port=8
  AIR_flow_rate : Display
  Compare To Zero : simulink/Logic and Bit Operations/Compare To Zero  relop=>  OutDataTypeStr=uint8
  Constant : Constant  Value=FC.R
  Constant1 : Constant  Value=FC.sel_UfH2
  Constant2 : Constant  Value=FC.sel_UfO2
  Gain : Gain
  H2 utilization Fuel flowrate : Fcn  Expr=60000*FC.Nc*u(2)*FC.R*u(5)/(FC.z*FC.F*u(4)*FC.Pstd*u(3)*u(1))
  H2_airflow1 : Display
  Mux1 : Mux  Inputs=5
  Mux5 : Mux  Inputs=5
  Mux6 : Mux  Inputs=2
  Mux7 : Mux  Inputs=2
  O2 utilization Air flowrate : Fcn  Expr=60000*FC.Nc*u(2)*FC.R*u(5)/(4*FC.F*u(4)*FC.Pstd*u(3)*u(1))
  P_air : Display
  P_fuel : Display
  Product2 : Product  RndMeth=Zero
  Saturation3 : Saturate  UpperLimit=inf  LowerLimit=FC.AirFr_Max*0.01
  Switch{1..4} (4 alike) : Switch  Criteria=u2 > Threshold  Threshold=0.5
  UF_H2 : Display
  UF_O2 : Display
  X : Display
  Y : Display
  i_current : Display
  i_current1 : Display
  i_current2 : Display
  Uf_H2 : Outport  VectorParamsAs1DForOutWhenUnconnected=off
  Uf_O2 : Outport  Port=2  VectorParamsAs1DForOutWhenUnconnected=off
  Fr_AirFuel : Outport  Port=3  VectorParamsAs1DForOutWhenUnconnected=off
  Uf_O2H2 : Outport  Port=4  VectorParamsAs1DForOutWhenUnconnected=off
  wires:
  Switch1/1 -> Mux7/2, UF_H2/1, Uf_H2/1
  Saturation3/1 -> Mux5/3
  Switch2/1 -> Mux7/1, UF_O2/1, Uf_O2/1  "Uf_O2"
  Gain/1 -> Fr_AirFuel/1
  Switch4/1 -> Mux6/1
  Switch3/1 -> Mux6/2
  Mux6/1 -> Gain/1
  Pf/1 -> P_fuel/1, Mux1/4
  T/1 -> i_current2/1, Mux1/5, Mux5/5
  O2 utilization Air flowrate/1 -> Switch4/1, Switch2/3
  Constant2/1 -> Switch2/2, Switch4/2
  Constant1/1 -> Switch3/2, Switch1/2
  H2 utilization Fuel flowrate/1 -> Switch3/1, Switch1/3
  i/1 -> i_current/1, Compare To Zero/1, Mux1/2, i_current1/1, Mux5/2
  Air/1 -> AIR_flow_rate/1, Switch2/1, Switch4/3, Saturation3/1
  y/1 -> Y/1, Mux5/1
  H2/1 -> H2_airflow1/1, Mux1/3, Switch1/1, Switch3/3
  x/1 -> X/1, Mux1/1
  Mux5/1 -> O2 utilization Air flowrate/1
  Mux1/1 -> H2 utilization Fuel flowrate/1
  Mux7/1 -> Product2/2
  Product2/1 -> Uf_O2H2/1
  Compare To Zero/1 -> Product2/1
  PAir/1 -> P_air/1, Mux5/4

== system Commande/fuzzy logic/Fuel Cell Stack1/Model/Discrete//Detailed/CellVoltage/Partial pressure ==
  in : Inport
  A2 : Fcn  Expr=(FC.R*u(1))/(2*FC.alpha*FC.F)
  Constant : Constant
  Cr : Fcn  Expr=(u(2)*FC.Pstd+u(3)*FC.Pstd)/(FC.R*u(1))
  Mux1 : Mux  Inputs=2
  Mux2 : Mux
  Nerst Voltage : Fcn  Expr=1.229+(u(1)-298.15)*(-44.43/(FC.z*FC.F))+(FC.R*u(1)/(FC.z*FC.F))*(log(u(2)*sqrt(u(3))/u(4)))
  PH2 : Fcn  Expr=u(3)*(1-u(2))*u(6)
  PH2O : Fcn  Expr=(FC.xy+2*u(5)*u(4))*u(7)
  PO2 : Fcn  Expr=u(5)*(1-u(4))*u(7)
  Saturation1 : Saturate  UpperLimit=inf  LowerLimit=0.0001
  Saturation4 : Saturate  UpperLimit=inf  LowerLimit=0.0001
  Saturation5 : Saturate  UpperLimit=inf  LowerLimit=0.0001
  Switch : Switch  Threshold=273+100
  Temp : Fcn  Expr=u(1)
  i0 calc : Fcn  Expr=2*FC.F*FC.k*u(1)*u(2)*exp(-FC.Dg/(FC.R*u(1)))/FC.h
  i0 : Outport  VectorParamsAs1DForOutWhenUnconnected=off
  A : Outport  Port=2  VectorParamsAs1DForOutWhenUnconnected=off
  Nerst : Outport  Port=3  VectorParamsAs1DForOutWhenUnconnected=off
  wires:
  Cr/1 -> Mux1/2
  Mux1/1 -> i0 calc/1
  in/1 -> PO2/1, PH2/1, Temp/1, PH2O/1
  Mux2/1 -> Cr/1, Nerst Voltage/1
  Constant/1 -> Switch/3
  Saturation5/1 -> Switch/1
  Switch/1 -> Mux2/4
  Saturation4/1 -> Mux2/3
  Saturation1/1 -> Mux2/2
  PH2/1 -> Saturation1/1
  PO2/1 -> Saturation4/1
  PH2O/1 -> Saturation5/1
  A2/1 -> A/1
  Nerst Voltage/1 -> Nerst/1
  i0 calc/1 -> i0/1
  Temp/1 -> Mux1/1, A2/1, Switch/2, Mux2/1

== system Commande/fuzzy logic/Fuel Cell Stack1/Model/Discrete//Detailed/CellVoltage/Uf calculator ==
  T : Inport
  x : Inport  Port=2
  y : Inport  Port=3
  Pf : Inport  Port=4
  PAir : Inport  Port=5
  H2 : Inport  Port=6
  Air : Inport  Port=7
  i : Inport  Port=8
  Compare To Zero : simulink/Logic and Bit Operations/Compare To Zero  relop=>  OutDataTypeStr=uint8
  Constant1 : Constant  Value=FC.sel_UfH2
  Constant2 : Constant  Value=FC.sel_UfO2
  Gain : Gain
  H2 utilization Fuel flowrate : Fcn  Expr=60000*FC.Nc*u(2)*FC.R*u(5)/(FC.z*FC.F*u(4)*FC.Pstd*u(3)*u(1))
  Mux1 : Mux  Inputs=5
  Mux5 : Mux  Inputs=5
  Mux6 : Mux  Inputs=2
  Mux7 : Mux  Inputs=2
  O2 utilization Air flowrate : Fcn  Expr=60000*FC.Nc*u(2)*FC.R*u(5)/(4*FC.F*u(4)*FC.Pstd*u(3)*u(1))
  Product2 : Product  RndMeth=Zero
  Saturation3 : Saturate  UpperLimit=inf  LowerLimit=FC.AirFr_Max*0.01
  Switch{1..4} (4 alike) : Switch  Criteria=u2 > Threshold  Threshold=0.5
  Uf_H2 : Outport  VectorParamsAs1DForOutWhenUnconnected=off
  Uf_O2 : Outport  Port=2  VectorParamsAs1DForOutWhenUnconnected=off
  Fr_AirFuel : Outport  Port=3  VectorParamsAs1DForOutWhenUnconnected=off
  Uf_O2H2 : Outport  Port=4  VectorParamsAs1DForOutWhenUnconnected=off
  wires:
  Compare To Zero/1 -> Product2/1
  Product2/1 -> Uf_O2H2/1
  Mux7/1 -> Product2/2
  Mux1/1 -> H2 utilization Fuel flowrate/1
  Mux5/1 -> O2 utilization Air flowrate/1
  x/1 -> Mux1/1
  H2/1 -> Switch3/3, Switch1/1, Mux1/3
  y/1 -> Mux5/1
  Air/1 -> Switch4/3, Switch2/1, Saturation3/1
  i/1 -> Mux5/2, Mux1/2, Compare To Zero/1
  H2 utilization Fuel flowrate/1 -> Switch1/3, Switch3/1
  Constant1/1 -> Switch1/2, Switch3/2
  Constant2/1 -> Switch2/2, Switch4/2
  O2 utilization Air flowrate/1 -> Switch2/3, Switch4/1
  T/1 -> Mux5/5, Mux1/5
  Pf/1 -> Mux1/4
  PAir/1 -> Mux5/4
  Mux6/1 -> Gain/1
  Switch3/1 -> Mux6/2
  Switch4/1 -> Mux6/1
  Gain/1 -> Fr_AirFuel/1
  Switch2/1 -> Uf_O2/1, Mux7/1  "Uf_O2"
  Saturation3/1 -> Mux5/3
  Switch1/1 -> Uf_H2/1, Mux7/2

== matlab function Commande/ML/ML Model/MATLAB Function ==
  data: T input; Vmpp output; Pfuel input; Pair input; Vfuel input; Vair input
function Vmpp = fcn(T, Pfuel, Pair, Vfuel, Vair)

    Vmpp = 0.0; % Predefine output as double to satisfy Simulink
    Vmpp = load_pytorch_model(T, Pfuel, Pair, Vfuel, Vair);
end
